simulink model "Noh_Nofusion"  (R2020b)
settings: Solver=FixedStepAuto  StartTime=0.0  StopTime=Inf  FixedStep=0.01  RelTol=1e-3
PostLoadFcn:
  | if any(exist('dsrtsu_mdlpostloadfcn', 'file') ~= 0), dsrtsu_mdlpostloadfcn('Execute', bdroot); end
InitFcn:
  | , if any(exist('rtifpga_mdlclblib', 'file') ~= 0), rtifpga_mdlclblib('Init', bdroot); end,
  | , if any(exist('dsmpb_private', 'file') ~= 0), dsmpb_private('dsmpb_mdlclblib', 'Init', bdroot); end,
undefined symbols (not defined in the file): ACC_TimeGap_DecSetSwt, ACC_TimeGap_IncSetSwt, AccelPedalPosn, AccelPedalPosnVldty, AccelPedlPosnDiagc, AccPedalOverride, ACU_ShiftInProgress, ADAS_Posn_CurLane, AESSwtReq, ALC_SwtReq, BrkPedalSts, CC_ACC_CANCEL_OFFSwt, CC_ACC_CRUISE_OFFSwt, CC_ACC_DecSetSpd_SetSwt, CC_ACC_IncSetSpd_ResuSwt, CC_ACCSwtErr, CharSpd_ms, CSA_NODE, CURRENT_GEAR, CurrentGearValid, DiscIntNeverNeededParam, DrvDoorSts, DrvSBR, DrvTrqReqOvld, ECMACCInterface, ECMRespACC, ELKSwtReq, EngLimpHomeSts, EngSpd, EngState, EngState_PHEV, EngTrqMaxActSpd, EngTrqMinAct, EPS_DrvInpTrqVal_HighReslolution, EPS_FailSts, EPS_LKATorqOvrlDlvd, EPS_LKATorqOvrlDlvdVld, EPS_LKATrqOvlDlvdSts, EPS_SteerMod, EPS_TrqSnsrSts, EQ4_APPINFO, EQ4_LA_ELEM, EQ4_LA_HDR, EQ4_LAP_ELEM, EQ4_LAP_HDR, EQ4_LH_ELEM, EQ4_LH_HDR, EQ4_LRE_ELEM, EQ4_LRE_HDR, ESS_PedSwtReq, ESS_VehSwtReq, FFogLmpSts_F_Pbox, FLWheelDriveDirection, FLWheelSpd, FrntWiprSwtSts, FrntWshrSwtSts, FRWheelDriveDirection, FRWheelSpd, HazardLmpSwtSts, HCU_AccelPedalPosn_Diag ... (+153)
libraries: simulink x132, dsmpblib x27
(part 8 of 14)

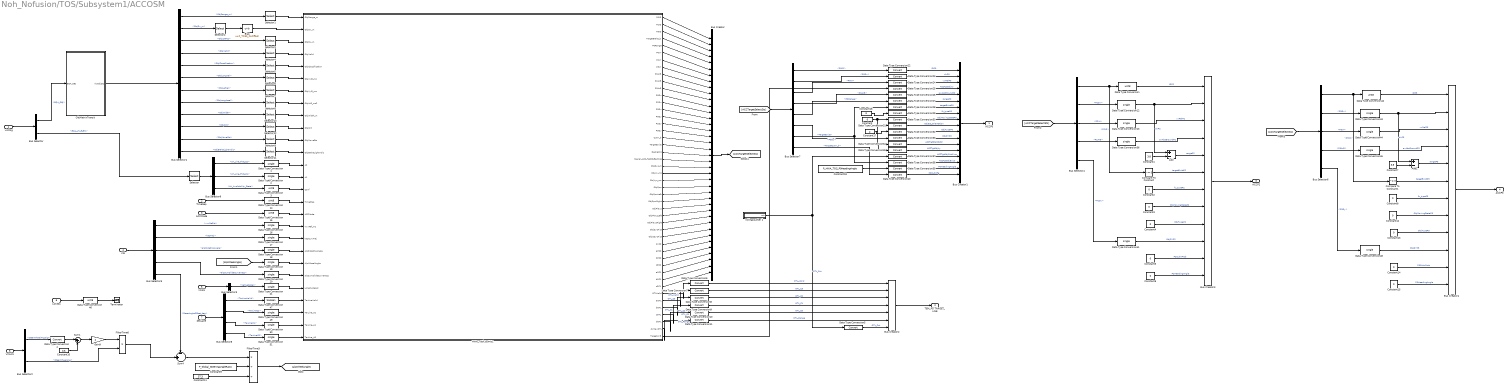
== system Noh_Nofusion/TOS/Subsystem1/ACCOSM ==
  visMsg : Inport
  TimeGap : Inport  Port=2
  ACCMode : Inport  Port=3
  VIE : Inport  Port=4
  VCAN : Inport  Port=5
  LCKSts : Inport  Port=6
  desLane : Inport  Port=7
  Add : Sum  Inputs=+-
  Add1 : Sum  Inputs=+-
  Bias : Bias  Bias=P_TOSS_DxOffset
  Bus Creator : BusCreator  Inputs=39
  Bus Creator1 : BusCreator  Inputs=18  OutDataTypeStr=Bus: TOS_ACCP0_BUS  NonVirtualBus=on
  Bus Creator2 : BusCreator  Inputs=7  OutDataTypeStr=Bus: TOS_P0_TARGET_LINE_BUS  NonVirtualBus=on
  Bus Creator3 : BusCreator  Inputs=12  OutDataTypeStr=Bus: TOS_ACCP2_BUS  NonVirtualBus=on
  Bus Creator4 : BusCreator  Inputs=12  OutDataTypeStr=Bus: TOS_ACCP3_BUS  NonVirtualBus=on
  Bus Selector : BusSelector  OutputSignals=EQ4_OBJ,EQ4_LH.EQ4_LH_ELEM
  Bus Selector4 : BusSelector  OutputSignals=P2ID,P2Dx,P2Vr,P2ArG,P2Dy
  Bus Selector6 : BusSelector  OutputSignals=P3ID,P3Dx,P3Vr,P3ArG,P3Dy
  Bus Selector7 : BusSelector  OutputSignals=P0ID,P0Dx,P0Vr,P0ArG,P0Range,P0Dy,TargetExist,TargetCutIn_b
  Bus Selector9 : BusSelector  OutputSignals=LH_Line_First_C2,LH_Line_First_C1,LH_Availability_State
  Bus Selector1 : BusSelector  OutputSignals=ObjRange_m,ObjDx_m,ObjLatPos,ObjValid,ObjClassification,ObjLongVel,ObjLatVel,ObjLongAccel,ObjWidth,ObjCnt,ObjMoveSts,ObjBrakeLightIndic
  Bus Selector2 : BusSelector  OutputSignals=CSA_NODE.CSA2_MSG.SteerWheelAngSign,CSA_NODE.CSA2_MSG.SteerWheelAng
  Bus Selector3 : BusSelector  OutputSignals=ABM_NODE.ABM2_MSG.VehLgtAccel
  Bus Selector5 : BusSelector  OutputSignals=vxvRefMs,kapTraj,alpSideSlipAngle,alpSumSlideCurveness,SteerAngleOffset_deg
  Bus Selector8 : BusSelector  OutputSignals=TarLineValid,TarLineC2,TarLineC1,TarLineC0
  Compare To Constant : simulink/Logic and Bit Operations/Compare To Constant  relop=~=  const=0  OutDataTypeStr=boolean
  Compare To Constant1 : simulink/Logic and Bit Operations/Compare To Constant  relop=~=  const=0  OutDataTypeStr=boolean
  Constant : Constant  Value=0
  Constant1 : Constant  Value=3.8  OutDataTypeStr=single
  Constant10 : Constant  Value=0.5  OutDataTypeStr=single
  Constant11 : Constant  Value=57.3  OutDataTypeStr=single
  Constant{2..4,8,12..13} (6 alike) : Constant  Value=0  OutDataTypeStr=uint8
  Constant{5..6,14..15} (4 alike) : Constant  Value=0  OutDataTypeStr=single
  Constant16 : Constant  Value=3
  Constant17 : Constant  Value=2
  Constant18 : Constant  Value=P_HWA_TOS_P0HeadingAngle
  Constant7 : Constant  Value=3.8  OutDataTypeStr=single
  Constant9 : Constant  Value=P_Global_SteeringAngleRatio
  Data Type Conversion{,3,14..15,42,46} (6 alike) : DataTypeConversion  OutDataTypeStr=uint8
  Data Type Conversion{1..2,12..13,16..21,36,41,43..45,48..51} (19 alike) : DataTypeConversion  OutDataTypeStr=single
  Data Type Conversion{4..11,22..35,37..40} (26 alike) : DataTypeConversion
  Data Type Conversion47 : DataTypeConversion  OutDataTypeStr=boolean
  FilterTime3 : Product  Inputs=*//  RndMeth=Zero
  FilterTime6 : Product  Inputs=**  RndMeth=Zero
  Gain9 : Gain  Gain=2
  HWA_Task100ms1 : Subsystem
  ObjMatrixTransit : Subsystem
  Selector : Selector  InputPortWidth=2  IndexOptions=Index vector (dialog)  Indices=1  OutputSizes=1
  Selector{1..12} (12 alike) : Selector  InputPortWidth=20  IndexOptions=Index vector (dialog)  Indices=[1:15]  OutputSizes=1
  Sum1 : Sum  Inputs=|-+
  Sum4 : Sum  Inputs=-+|
  Terminator : Terminator
  VCAN1 : InportShadow  Port=5
  rollingcounter 1 : Subsystem
  ACCP0 : Outport  OutDataTypeStr=Bus: TOS_ACCP0_BUS
  TEM_P0_TARGET_LINE : Outport  Port=2  OutDataTypeStr=Bus: TOS_P0_TARGET_LINE_BUS  PortDimensions=1  BusOutputAsStruct=on
  ACCP2 : Outport  Port=3  OutDataTypeStr=Bus: TOS_ACCP2_BUS
  ACCP3 : Outport  Port=4  OutDataTypeStr=Bus: TOS_ACCP3_BUS
  wires:
  Data Type Conversion51/1 -> HWA_Task100ms1/27(TarLine_A0)
  Data Type Conversion46/1 -> Terminator/1
  Constant18/1 -> Data Type Conversion39/1
  HWA_Task100ms1/46(TargetVyG) -> Data Type Conversion25/1
  Constant17/1 -> Data Type Conversion32/1
  Constant16/1 -> Data Type Conversion29/1
  Selector2/1 -> Bias/1
  [ACCTargetSelectSts] -> Bus Selector6/1
  Bus Selector6/1 -> Compare To Constant1/1, Data Type Conversion42/1  "<P3ID>"
  Data Type Conversion42/1 -> Bus Creator4/1  "IDP3"
  Bus Selector6/2 -> Data Type Conversion43/1  "<P3Dx>"
  Data Type Conversion43/1 -> Add1/1, Bus Creator4/2  "dxP3"
  Bus Selector6/3 -> Data Type Conversion44/1  "<P3Vr>"
  Data Type Conversion44/1 -> Bus Creator4/3  "vxRelP3"
  Bus Selector6/4 -> Data Type Conversion45/1  "<P3ArG>"
  Data Type Conversion45/1 -> Bus Creator4/4  "axAbsGroundP3"
  Add1/1 -> Bus Creator4/5  "rangeP3"
  Constant7/1 -> Add1/2
  Compare To Constant1/1 -> Bus Creator4/6  "targetExistP3"
  Constant8/1 -> Bus Creator4/7  "fu_typeP3"
  Constant12/1 -> Bus Creator4/8  "ObjMovingStateP3"
  Constant13/1 -> Bus Creator4/9  "ObjTypeP3"
  Bus Selector6/5 -> Data Type Conversion48/1  "<P3Dy>"
  Data Type Conversion48/1 -> Bus Creator4/10  "ObjDYP3"
  Constant14/1 -> Bus Creator4/11  "P3CutinProb"
  Constant15/1 -> Bus Creator4/12  "P3HeadingAngle"
  Bus Creator4/1 -> ACCP3/1
  Bus Creator3/1 -> ACCP2/1
  Constant6/1 -> Bus Creator3/12  "P2HeadingAngle"
  Constant5/1 -> Bus Creator3/11  "P2CutinProb"
  Data Type Conversion41/1 -> Bus Creator3/10  "ObjDYP2"
  Bus Selector4/5 -> Data Type Conversion41/1  "<P2Dy>"
  Constant4/1 -> Bus Creator3/9  "ObjTypeP2"
  Constant3/1 -> Bus Creator3/8  "ObjMovingStateP2"
  Constant2/1 -> Bus Creator3/7  "fu_typeP2"
  Compare To Constant/1 -> Bus Creator3/6  "targetExistP2"
  Constant1/1 -> Add/2
  Add/1 -> Bus Creator3/5  "rangeP2"
  Data Type Conversion36/1 -> Bus Creator3/4  "axAbsGroundP2"
  Bus Selector4/4 -> Data Type Conversion36/1  "<P2ArG>"
  Data Type Conversion13/1 -> Bus Creator3/3  "vxRelP2"
  Bus Selector4/3 -> Data Type Conversion13/1  "<P2Vr>"
  Data Type Conversion12/1 -> Bus Creator3/2, Add/1  "dxP2"
  Bus Selector4/2 -> Data Type Conversion12/1  "<P2Dx>"
  Data Type Conversion/1 -> Bus Creator3/1  "IDP2"
  Bus Selector4/1 -> Data Type Conversion/1, Compare To Constant/1  "<P2ID>"
  [ACCTargetSelectSts] -> Bus Selector4/1
  ObjMatrixTransit/1(VisObjSts) -> Bus Selector1/1
  Bus Selector/1 -> ObjMatrixTransit/1(EQ4_OBJ)  "<EQ4_OBJ>"
  Selector12/1 -> HWA_Task100ms1/10(ObjCnt)
  Selector11/1 -> HWA_Task100ms1/12(ObjBrakeLightIndic)
  Selector10/1 -> HWA_Task100ms1/9(ObjWidth_m)
  Selector9/1 -> HWA_Task100ms1/11(ObjMoveSts)
  Selector8/1 -> HWA_Task100ms1/8(ObjArG_ms2)
  Selector7/1 -> HWA_Task100ms1/7(ObjVyG_ms)
  Selector6/1 -> HWA_Task100ms1/6(ObjVxG_ms)
  Selector5/1 -> HWA_Task100ms1/5(ObjClassification)
  Selector4/1 -> HWA_Task100ms1/4(ObjValid)
  Selector3/1 -> HWA_Task100ms1/3(ObjDy_m)
  Bias/1 -> HWA_Task100ms1/2(ObjDx_m)
  Selector1/1 -> HWA_Task100ms1/1(ObjRange_m)
  Selector/1 -> Bus Selector9/1
  Bus Selector/2 -> Selector/1  "<EQ4_LH_ELEM>"
  visMsg/1 -> Bus Selector/1
  Data Type Conversion11/1 -> Bus Creator2/6  "OTL_Range"
  Data Type Conversion10/1 -> Bus Creator2/5  "OTL_C0"
  Data Type Conversion9/1 -> Bus Creator2/4  "OTL_C1"
  Data Type Conversion8/1 -> Bus Creator2/3  "OTL_C2"
  Data Type Conversion7/1 -> Bus Creator2/2  "OTL_C3"
  Data Type Conversion6/1 -> Bus Creator2/1  "OTL_Valid"
  Data Type Conversion5/1 -> Bus Creator2/7  "OTL_Cnt"
  Bus Creator2/1 -> TEM_P0_TARGET_LINE/1
  HWA_Task100ms1/42(bOTL) -> Data Type Conversion8/1  "OTL_C2"
  HWA_Task100ms1/41(aOTL) -> Data Type Conversion7/1  "OTL_C3"
  HWA_Task100ms1/40(OTLValid) -> Data Type Conversion6/1  "OTL_Valid"
  HWA_Task100ms1/43(cOTL) -> Data Type Conversion9/1  "OTL_C1"
  rollingcounter 1/1(cnt) -> Data Type Conversion5/1, Data Type Conversion37/1  "OTL_Cnt"
  HWA_Task100ms1/45(dxMaxOTL) -> Data Type Conversion11/1  "OTL_Range"
  HWA_Task100ms1/44(dOTL) -> Data Type Conversion10/1  "OTL_C0"
  Data Type Conversion4/1 -> Sum1/1
  Bus Selector2/2 -> FilterTime6/2  "<SteerWheelAng>"
  Bus Selector2/1 -> Data Type Conversion4/1  "<SteerWheelAngSign>"
  Sum1/1 -> Gain9/1
  Gain9/1 -> FilterTime6/1
  Constant10/1 -> Sum1/2
  VCAN1/1 -> Bus Selector2/1
  Constant9/1 -> FilterTime3/2
  Bus Selector5/5 -> Sum4/1  "<SteerAngleOffset_deg>"
  FilterTime3/1 -> [alpWheelAngle]
  Sum4/1 -> FilterTime3/1
  Constant11/1 -> FilterTime3/3
  FilterTime6/1 -> Sum4/2
  HWA_Task100ms1/34(aPC0) -> Bus Creator/34
  HWA_Task100ms1/38(bPC1) -> Bus Creator/38
  Bus Selector7/1 -> Data Type Conversion22/1  "<P0ID>"
  Data Type Conversion3/1 -> HWA_Task100ms1/15(Conf)
  Data Type Conversion22/1 -> Bus Creator1/1  "IDP0"
  Data Type Conversion27/1 -> Bus Creator1/6  "rangeP0"
  Data Type Conversion1/1 -> HWA_Task100ms1/13(A2)
  HWA_Task100ms1/2(P2ID) -> Bus Creator/2
  Data Type Conversion2/1 -> HWA_Task100ms1/14(A1)
  Data Type Conversion37/1 -> Bus Creator1/15  "ACCTgtObjCntAlive"
  HWA_Task100ms1/1(P0ID) -> Bus Creator/1
  Bus Selector3/1 -> Data Type Conversion21/1  "<VehLgtAccel>"
  Bus Selector1/9 -> Selector10/1  "<ObjWidth>"
  Data Type Conversion19/1 -> HWA_Task100ms1/21(AlpWheelAngle)
  Bus Selector7/3 -> Data Type Conversion24/1  "<P0Vr>"
  Bus Selector9/1 -> Data Type Conversion1/1  "<LH_Line_First_C2>"
  VIE/1 -> Bus Selector5/1
  Data Type Conversion38/1 -> Bus Creator1/16  "ACCTgtObjExist"
  Bus Selector7/6 -> Data Type Conversion33/1  "<P0Dy>"
  Bus Selector7/2 -> Data Type Conversion23/1  "<P0Dx>"
  Data Type Conversion29/1 -> Bus Creator1/8  "fu_typeP0"
  Bus Selector7/8 -> Data Type Conversion40/1  "<TargetCutIn_b>"
  HWA_Task100ms1/32(ObjqDycHist) -> Bus Creator/32
  Data Type Conversion32/1 -> Bus Creator1/11  "ObjTypeP0"
  Data Type Conversion35/1 -> Bus Creator1/14  "ACCTgtObjAy"
  VCAN/1 -> Bus Selector3/1
  Data Type Conversion34/1 -> Bus Creator1/13  "ACCTgtObjObstcl"
  Bus Selector8/1 -> Data Type Conversion47/1  "<TarLineValid>"
  Bus Selector5/1 -> Data Type Conversion16/1  "<vxvRefMs>"
  Data Type Conversion17/1 -> HWA_Task100ms1/19(kapCurvTraj)
  Data Type Conversion28/1 -> Bus Creator1/7  "targetExistP0"
  Bus Selector1/7 -> Selector7/1  "<ObjLatVel>"
  HWA_Task100ms1/8(P3Vr) -> Bus Creator/8
  Bus Selector1/8 -> Selector8/1  "<ObjLongAccel>"
  Data Type Conversion49/1 -> HWA_Task100ms1/25(TarLine_A2)
  ACCMode/1 -> Data Type Conversion15/1
  HWA_Task100ms1/22(ObjDyc_m) -> Bus Creator/22
  Data Type Conversion18/1 -> HWA_Task100ms1/20(AlpSideSlipAngle)
  Data Type Conversion30/1 -> Bus Creator1/9  "ObjMovingStateP0"
  HWA_Task100ms1/11(P3ArG) -> Bus Creator/11
  Data Type Conversion25/1 -> Bus Creator1/4  "ACCTgtObjVy"
  TimeGap/1 -> Data Type Conversion14/1
  Data Type Conversion23/1 -> Bus Creator1/2  "dxP0"
  Data Type Conversion21/1 -> HWA_Task100ms1/23(LongitudeAcc)
  Bus Creator/1 -> [ACCTargetSelectSts]
  HWA_Task100ms1/31(ObjDycHist) -> Bus Creator/31
  Bus Selector1/5 -> Selector5/1  "<ObjClassification>"
  Bus Selector7/5 -> Data Type Conversion27/1  "<P0Range>"
  Bus Selector5/2 -> Data Type Conversion17/1  "<kapTraj>"
  Bus Selector1/3 -> Selector3/1  "<ObjLatPos>"
  Constant/1 -> Data Type Conversion30/1, Data Type Conversion31/1, Data Type Conversion34/1, Data Type Conversion35/1
  Data Type Conversion47/1 -> HWA_Task100ms1/24(TarLineValid)
  HWA_Task100ms1/4(TargetBrake_b) -> Bus Creator/4
  Data Type Conversion14/1 -> HWA_Task100ms1/16(TimeGap)
  HWA_Task100ms1/15(P0Dy) -> Bus Creator/15
  HWA_Task100ms1/33(dxC0) -> Bus Creator/33
  Data Type Conversion39/1 -> Bus Creator1/17  "P0HeadingAngle"
  HWA_Task100ms1/21(Signal_ACC_TgtObjBarDisp) -> Bus Creator/21
  HWA_Task100ms1/24(ObjVyc_ms) -> Bus Creator/24
  HWA_Task100ms1/16(P2Dy) -> Bus Creator/16
  Bus Selector8/3 -> Data Type Conversion50/1  "<TarLineC1>"
  HWA_Task100ms1/30(ObjPlausRight) -> Bus Creator/30
  HWA_Task100ms1/13(P2Dx) -> Bus Creator/13
  Bus Selector1/11 -> Selector9/1  "<ObjMoveSts>"
  HWA_Task100ms1/35(bPC0) -> Bus Creator/35
  Data Type Conversion16/1 -> HWA_Task100ms1/18(VxvRef_ms)
  Bus Selector9/2 -> Data Type Conversion2/1  "<LH_Line_First_C1>"
  HWA_Task100ms1/18(CutIn_b) -> Bus Creator/18
  HWA_Task100ms1/27(ObjSpwRight) -> Bus Creator/27
  [ACCTargetSelectSts] -> Bus Selector7/1
  HWA_Task100ms1/3(P3ID) -> Bus Creator/3
  HWA_Task100ms1/20(DesireDis) -> Bus Creator/20
  Bus Selector7/4 -> Data Type Conversion26/1  "<P0ArG>"
  Data Type Conversion31/1 -> Bus Creator1/10  "Object_Orientation"
  Data Type Conversion50/1 -> HWA_Task100ms1/26(TarLine_A1)
  Bus Selector1/1 -> Selector1/1  "<ObjRange_m>"
  Bus Selector1/6 -> Selector6/1  "<ObjLongVel>"
  Bus Selector1/12 -> Selector11/1  "<ObjBrakeLightIndic>"
  Bus Selector5/3 -> Data Type Conversion18/1  "<alpSideSlipAngle>"
  HWA_Task100ms1/14(P3Dx) -> Bus Creator/14
  Data Type Conversion33/1 -> Bus Creator1/12  "ObjDYP0"
  Bus Selector5/4 -> Data Type Conversion20/1  "<alpSumSlideCurveness>"
  HWA_Task100ms1/9(P0ArG) -> Bus Creator/9
  HWA_Task100ms1/36(cPC0) -> Bus Creator/36
  HWA_Task100ms1/39(cPC1) -> Bus Creator/39
  HWA_Task100ms1/12(P0Dx) -> Bus Creator/12
  HWA_Task100ms1/17(P3Dy) -> Bus Creator/17
  HWA_Task100ms1/19(TargetExist) -> Bus Creator/19
  Bus Selector1/10 -> Selector12/1  "<ObjCnt>"
  HWA_Task100ms1/10(P2ArG) -> Bus Creator/10
  HWA_Task100ms1/26(ObjSpwLeft) -> Bus Creator/26
  HWA_Task100ms1/37(aPC1) -> Bus Creator/37
  HWA_Task100ms1/5(P0Range) -> Bus Creator/5
  Data Type Conversion26/1 -> Bus Creator1/5  "axAbsGroundP0"
  Bus Selector1/2 -> Selector2/1  "<ObjDx_m>"
  HWA_Task100ms1/28(ObjPlaus) -> Bus Creator/28
  LCKSts/1 -> Data Type Conversion46/1
  Data Type Conversion24/1 -> Bus Creator1/3  "vxRelP0"
  Bus Selector8/2 -> Data Type Conversion49/1  "<TarLineC2>"
  Bus Selector1/4 -> Selector4/1  "<ObjValid>"
  HWA_Task100ms1/7(P2Vr) -> Bus Creator/7
  HWA_Task100ms1/29(ObjPlausLeft) -> Bus Creator/29
  Data Type Conversion40/1 -> Bus Creator1/18  "P0CutInflg"
  desLane/1 -> Bus Selector8/1
  Bus Selector9/3 -> Data Type Conversion3/1  "<LH_Availability_State>"
  [alpWheelAngle] -> Data Type Conversion19/1
  HWA_Task100ms1/25(ObjSpw) -> Bus Creator/25
  HWA_Task100ms1/6(P0Vr) -> Bus Creator/6
  Bus Selector7/7 -> Data Type Conversion38/1, Data Type Conversion28/1  "<TargetExist>"
  Data Type Conversion15/1 -> HWA_Task100ms1/17(ACCMode)
  HWA_Task100ms1/23(ObjVy_ms) -> Bus Creator/23
  Data Type Conversion20/1 -> HWA_Task100ms1/22(alpSumSlideCurveness)
  Bus Selector8/4 -> Data Type Conversion51/1  "<TarLineC0>"
  Bus Creator1/1 -> ACCP0/1

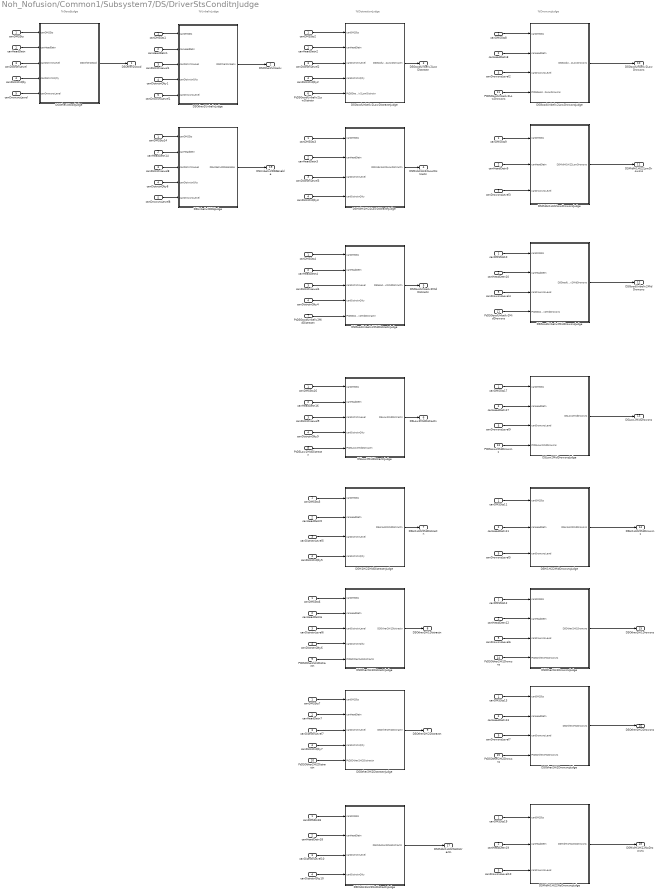
== system Noh_Nofusion/Common1/Subsystem7/DS/DriverStsConditnJudge ==
  note: %DrowsnsJudge
  note: %DistractionJudge
  note: %UnbelivJudge
  note: %GoodJudge
  canDMSSts : Inport
  canHeadDetn : Inport  Port=2
  canDistrctnLevel : Inport  Port=3
  canDistrctnQlty : Inport  Port=4
  canDrowsnsLevel : Inport  Port=5
  PtDSGoodUnbeliv2LowDistrctn : Inport  Port=6
  PtDSGoodUnbeliv2MidDistractn : Inport  Port=7
  PtDSLow2MidDistractn : Inport  Port=8
  PtDSOther2Hi1Distractn : Inport  Port=9
  PtDSOther2Hi2Distractn : Inport  Port=10
  PtDSGoodUnbeliv2LowDrowsns : Inport  Port=11
  PtDSGoodUnbeliv2MidDrowsns : Inport  Port=12
  PtDSLow2MidDrowsns : Inport  Port=13
  PtDSOther2Hi1Drowsns : Inport  Port=14
  PtDSOther2Hi2Drowsns : Inport  Port=15
  DSGoodUnbeliv2LowDistractnJudge : Subsystem
  DSGoodUnbeliv2LowDrowsnsJudge : Subsystem
  DSGoodUnbeliv2MidDistractnJudge : Subsystem
  DSGoodUnbeliv2MidDrowsnsJudge : Subsystem
  DSHi1Hi22MidDistractnJudge : Subsystem
  DSHi1Hi22MidDrowsnsJudge : Subsystem
  DSLow2MidDistractnJudge : Subsystem
  DSLow2MidDrowsnsJudge : Subsystem
  DSMidHi1Hi22LowDistractnJudge : Subsystem
  DSMidHi1Hi22LowDrowsnsJudge : Subsystem
  DSMidHi1Hi22NoDistractnJudge : Subsystem
  DSMidHi1Hi22NoDrowsnsJudge : Subsystem
  DSOther2GoodJudge : Subsystem
  DSOther2Hi1DistractnJudge : Subsystem
  DSOther2Hi1DrowsnsJudge : Subsystem
  DSOther2Hi2DistractnJudge : Subsystem
  DSOther2Hi2DrowsnsJudge : Subsystem
  DSOther2UnbelivJudge : Subsystem
  DSUnbeliv2DDAJudge : Subsystem
  canDMSSts{1..14,16..19} (18 alike) : InportShadow
  canDistrctnLevel{1..10} (10 alike) : InportShadow  Port=3
  canDistrctnQlty{1..10} (10 alike) : InportShadow  Port=4
  canDrowsnsLevel{1..10} (10 alike) : InportShadow  Port=5
  canHeadDetn{1..14,16..19} (18 alike) : InportShadow  Port=2
  DSOther2Good : Outport
  DSOther2Unbeliv : Outport  Port=2
  DSGoodUnbeliv2LowDistractn : Outport  Port=3
  DSMidHi1Hi22LowDistractn : Outport  Port=4
  DSGoodUnbeliv2MidDistractn : Outport  Port=5
  DSLow2MidDistractn : Outport  Port=6
  DSHi1Hi22MidDistractn : Outport  Port=7
  DSOther2Hi1Distractn : Outport  Port=8
  DSOther2Hi2Distractn : Outport  Port=9
  DSGoodUnbeliv2LowDrowsns : Outport  Port=10
  DSMidHi1Hi22LowDrowsns : Outport  Port=11
  DSGoodUnbeliv2MidDrowsns : Outport  Port=12
  DSLow2MidDrowsns : Outport  Port=13
  DSHi1Hi22MidDrowsns : Outport  Port=14
  DSOther2Hi1Drowsns : Outport  Port=15
  DSOther2Hi2Drowsns : Outport  Port=16
  DSMidHi1Hi22NoDistractn : Outport  Port=17
  DSMidHi1Hi22NoDrowsns : Outport  Port=18
  DSUnbeliv2DDAEnable : Outport  Port=19
  wires:
  PtDSOther2Hi2Drowsns/1 -> DSOther2Hi2DrowsnsJudge/4(PtDSOther2Hi2Drowsns)
  PtDSOther2Hi1Drowsns/1 -> DSOther2Hi1DrowsnsJudge/4(PtDSOther2Hi1Drowsns)
  PtDSLow2MidDrowsns/1 -> DSLow2MidDrowsnsJudge/4(PtDSLow2MidDrowsns)
  PtDSGoodUnbeliv2MidDrowsns/1 -> DSGoodUnbeliv2MidDrowsnsJudge/4(PtDSGoodUnbeliv2MidDrowsns)
  PtDSGoodUnbeliv2LowDrowsns/1 -> DSGoodUnbeliv2LowDrowsnsJudge/4(PtDSGoodUnbeliv2LowDrowsns)
  PtDSOther2Hi2Distractn/1 -> DSOther2Hi2DistractnJudge/5(PtDSOther2Hi2Distractn)
  PtDSOther2Hi1Distractn/1 -> DSOther2Hi1DistractnJudge/5(PtDSOther2Hi1Distractn)
  PtDSLow2MidDistractn/1 -> DSLow2MidDistractnJudge/5(PtDSLow2MidDistractn)
  PtDSGoodUnbeliv2MidDistractn/1 -> DSGoodUnbeliv2MidDistractnJudge/5(PtDSGoodUnbeliv2MidDistractn)
  PtDSGoodUnbeliv2LowDistrctn/1 -> DSGoodUnbeliv2LowDistractnJudge/5(PtDSGoodUnbeliv2LowDistrctn)
  DSUnbeliv2DDAJudge/1(DSUnbeliv2DDAEnable) -> DSUnbeliv2DDAEnable/1
  canDMSSts14/1 -> DSUnbeliv2DDAJudge/1(canDMSSts)
  canHeadDetn14/1 -> DSUnbeliv2DDAJudge/2(canHeadDetn)
  canDistrctnLevel8/1 -> DSUnbeliv2DDAJudge/3(canDistrctnLevel)
  canDistrctnQlty8/1 -> DSUnbeliv2DDAJudge/4(canDistrctnQlty)
  canDrowsnsLevel8/1 -> DSUnbeliv2DDAJudge/5(canDrowsnsLevel)
  DSMidHi1Hi22NoDrowsnsJudge/1(DSMidHi1Hi22NoDrowsns) -> DSMidHi1Hi22NoDrowsns/1
  canDMSSts19/1 -> DSMidHi1Hi22NoDrowsnsJudge/1(canDMSSts)
  canHeadDetn19/1 -> DSMidHi1Hi22NoDrowsnsJudge/2(canHeadDetn)
  canDrowsnsLevel10/1 -> DSMidHi1Hi22NoDrowsnsJudge/3(canDrowsnsLevel)
  DSMidHi1Hi22NoDistractnJudge/1(DSMidHi1Hi22NoDistractn) -> DSMidHi1Hi22NoDistractn/1
  canDMSSts18/1 -> DSMidHi1Hi22NoDistractnJudge/1(canDMSSts)
  canHeadDetn18/1 -> DSMidHi1Hi22NoDistractnJudge/2(canHeadDetn)
  canDistrctnLevel10/1 -> DSMidHi1Hi22NoDistractnJudge/3(canDistrctnLevel)
  canDistrctnQlty10/1 -> DSMidHi1Hi22NoDistractnJudge/4(canDistrctnQlty)
  DSLow2MidDrowsnsJudge/1(DSLow2MidDrowsns) -> DSLow2MidDrowsns/1
  canDMSSts17/1 -> DSLow2MidDrowsnsJudge/1(canDMSSts)
  canHeadDetn17/1 -> DSLow2MidDrowsnsJudge/2(canHeadDetn)
  canDrowsnsLevel9/1 -> DSLow2MidDrowsnsJudge/3(canDrowsnsLevel)
  canDMSSts16/1 -> DSLow2MidDistractnJudge/1(canDMSSts)
  canHeadDetn16/1 -> DSLow2MidDistractnJudge/2(canHeadDetn)
  canDistrctnLevel9/1 -> DSLow2MidDistractnJudge/3(canDistrctnLevel)
  canDistrctnQlty9/1 -> DSLow2MidDistractnJudge/4(canDistrctnQlty)
  DSLow2MidDistractnJudge/1(DSLow2MidDistractn) -> DSLow2MidDistractn/1
  DSOther2Hi2DrowsnsJudge/1(DSOther2Hi2Drowsns) -> DSOther2Hi2Drowsns/1
  canDMSSts13/1 -> DSOther2Hi2DrowsnsJudge/1(canDMSSts)
  canHeadDetn13/1 -> DSOther2Hi2DrowsnsJudge/2(canHeadDetn)
  canDrowsnsLevel7/1 -> DSOther2Hi2DrowsnsJudge/3(canDrowsnsLevel)
  DSOther2Hi1DrowsnsJudge/1(DSOther2Hi1Drowsns) -> DSOther2Hi1Drowsns/1
  canDrowsnsLevel6/1 -> DSOther2Hi1DrowsnsJudge/3(canDrowsnsLevel)
  canHeadDetn12/1 -> DSOther2Hi1DrowsnsJudge/2(canHeadDetn)
  canDMSSts12/1 -> DSOther2Hi1DrowsnsJudge/1(canDMSSts)
  canDMSSts11/1 -> DSHi1Hi22MidDrowsnsJudge/1(canDMSSts)
  canHeadDetn11/1 -> DSHi1Hi22MidDrowsnsJudge/2(canHeadDetn)
  canDrowsnsLevel5/1 -> DSHi1Hi22MidDrowsnsJudge/3(canDrowsnsLevel)
  DSHi1Hi22MidDrowsnsJudge/1(DSHi1Hi22MidDrowsns) -> DSHi1Hi22MidDrowsns/1
  DSGoodUnbeliv2MidDrowsnsJudge/1(DSGoodUnbeliv2MidDrowsns) -> DSGoodUnbeliv2MidDrowsns/1
  canDrowsnsLevel4/1 -> DSGoodUnbeliv2MidDrowsnsJudge/3(canDrowsnsLevel)
  canHeadDetn10/1 -> DSGoodUnbeliv2MidDrowsnsJudge/2(canHeadDetn)
  canDMSSts10/1 -> DSGoodUnbeliv2MidDrowsnsJudge/1(canDMSSts)
  canDrowsnsLevel3/1 -> DSMidHi1Hi22LowDrowsnsJudge/3(canDrowsnsLevel)
  canHeadDetn9/1 -> DSMidHi1Hi22LowDrowsnsJudge/2(canHeadDetn)
  canDMSSts9/1 -> DSMidHi1Hi22LowDrowsnsJudge/1(canDMSSts)
  DSMidHi1Hi22LowDrowsnsJudge/1(DSMidHi1Hi22LowDrowsns) -> DSMidHi1Hi22LowDrowsns/1
  canDrowsnsLevel2/1 -> DSGoodUnbeliv2LowDrowsnsJudge/3(canDrowsnsLevel)
  canHeadDetn8/1 -> DSGoodUnbeliv2LowDrowsnsJudge/2(canHeadDetn)
  canDMSSts8/1 -> DSGoodUnbeliv2LowDrowsnsJudge/1(canDMSSts)
  DSGoodUnbeliv2LowDrowsnsJudge/1(DSGoodUnbeliv2LowDrowsns) -> DSGoodUnbeliv2LowDrowsns/1
  canDistrctnQlty7/1 -> DSOther2Hi2DistractnJudge/4(canDistrctnQlty)
  canDistrctnLevel7/1 -> DSOther2Hi2DistractnJudge/3(canDistrctnLevel)
  canHeadDetn7/1 -> DSOther2Hi2DistractnJudge/2(canHeadDetn)
  canDMSSts7/1 -> DSOther2Hi2DistractnJudge/1(canDMSSts)
  DSOther2Hi2DistractnJudge/1(DSOther2Hi2Distractn) -> DSOther2Hi2Distractn/1
  canDistrctnQlty6/1 -> DSOther2Hi1DistractnJudge/4(canDistrctnQlty)
  canDistrctnLevel6/1 -> DSOther2Hi1DistractnJudge/3(canDistrctnLevel)
  canHeadDetn6/1 -> DSOther2Hi1DistractnJudge/2(canHeadDetn)
  canDMSSts6/1 -> DSOther2Hi1DistractnJudge/1(canDMSSts)
  DSOther2Hi1DistractnJudge/1(DSOther2Hi1Distractn) -> DSOther2Hi1Distractn/1
  DSHi1Hi22MidDistractnJudge/1(DSHi1Hi22MidDistractn) -> DSHi1Hi22MidDistractn/1
  canDistrctnQlty5/1 -> DSHi1Hi22MidDistractnJudge/4(canDistrctnQlty)
  canDistrctnLevel5/1 -> DSHi1Hi22MidDistractnJudge/3(canDistrctnLevel)
  canHeadDetn5/1 -> DSHi1Hi22MidDistractnJudge/2(canHeadDetn)
  canDMSSts5/1 -> DSHi1Hi22MidDistractnJudge/1(canDMSSts)
  DSGoodUnbeliv2MidDistractnJudge/1(DSGoodUnbeliv2MidDistractn) -> DSGoodUnbeliv2MidDistractn/1
  canDistrctnQlty4/1 -> DSGoodUnbeliv2MidDistractnJudge/4(canDistrctnQlty)
  canDistrctnLevel4/1 -> DSGoodUnbeliv2MidDistractnJudge/3(canDistrctnLevel)
  canHeadDetn4/1 -> DSGoodUnbeliv2MidDistractnJudge/2(canHeadDetn)
  canDMSSts4/1 -> DSGoodUnbeliv2MidDistractnJudge/1(canDMSSts)
  DSMidHi1Hi22LowDistractnJudge/1(DSMidHi1Hi22LowDistractn) -> DSMidHi1Hi22LowDistractn/1
  canDistrctnQlty3/1 -> DSMidHi1Hi22LowDistractnJudge/4(canDistrctnQlty)
  canDistrctnLevel3/1 -> DSMidHi1Hi22LowDistractnJudge/3(canDistrctnLevel)
  canHeadDetn3/1 -> DSMidHi1Hi22LowDistractnJudge/2(canHeadDetn)
  canDMSSts3/1 -> DSMidHi1Hi22LowDistractnJudge/1(canDMSSts)
  canDistrctnQlty2/1 -> DSGoodUnbeliv2LowDistractnJudge/4(canDistrctnQlty)
  canDistrctnLevel2/1 -> DSGoodUnbeliv2LowDistractnJudge/3(canDistrctnLevel)
  canHeadDetn2/1 -> DSGoodUnbeliv2LowDistractnJudge/2(canHeadDetn)
  canDMSSts2/1 -> DSGoodUnbeliv2LowDistractnJudge/1(canDMSSts)
  DSGoodUnbeliv2LowDistractnJudge/1(DSGoodUnbeliv2LowDistractn) -> DSGoodUnbeliv2LowDistractn/1
  DSOther2UnbelivJudge/1(DSOther2Unbeliv) -> DSOther2Unbeliv/1
  canDrowsnsLevel1/1 -> DSOther2UnbelivJudge/5(canDrowsnsLevel)
  canDistrctnQlty1/1 -> DSOther2UnbelivJudge/4(canDistrctnQlty)
  canDistrctnLevel1/1 -> DSOther2UnbelivJudge/3(canDistrctnLevel)
  canHeadDetn1/1 -> DSOther2UnbelivJudge/2(canHeadDetn)
  canDMSSts1/1 -> DSOther2UnbelivJudge/1(canDMSSts)
  canDrowsnsLevel/1 -> DSOther2GoodJudge/5(canDrowsnsLevel)
  canDistrctnQlty/1 -> DSOther2GoodJudge/4(canDistrctnQlty)
  canDistrctnLevel/1 -> DSOther2GoodJudge/3(canDistrctnLevel)
  canHeadDetn/1 -> DSOther2GoodJudge/2(canHeadDetn)
  DSOther2GoodJudge/1(DSOther2Good) -> DSOther2Good/1
  canDMSSts/1 -> DSOther2GoodJudge/1(canDMSSts)

== system Noh_Nofusion/Subsystem2/ACCOSM/HWA_Task100ms1/OTL1 ==
  vRef : Inport
  tCycle : Inport  Port=2
  tSameHandle : Inport  Port=3
  CutIn : Inport  Port=4
  P0Dx : Inport  Port=5
  P0Dy : Inport  Port=6
  EgoDDeltaX : Inport  Port=7
  EgoDDeltaY : Inport  Port=8
  EgoCosOfPsi : Inport  Port=9
  EgoSinOfPsi : Inport  Port=10
  Memory31 : Memory  InitialCondition=zeros(24,1)  InheritSampleTime=on
  Memory32 : Memory  InitialCondition=zeros(24,1)  InheritSampleTime=on
  Memory33 : Memory  InitialCondition=uint8(0)  InheritSampleTime=on
  P0TrajHistCalc01 : MATLAB Function  TreatAsAtomicUnit=on
  P0TrajHistCalc1 : MATLAB Function  TreatAsAtomicUnit=on
  Terminator : Terminator
  Terminator1 : Terminator
  Terminator2 : Terminator
  LineValid : Outport
  a : Outport  Port=2
  b : Outport  Port=3
  c : Outport  Port=4
  d : Outport  Port=5
  dxMin : Outport  Port=6
  dxMax : Outport  Port=7
  wires:
  vRef/1 -> P0TrajHistCalc01/1(vRef)
  CutIn/1 -> P0TrajHistCalc01/4(CutIn)
  P0TrajHistCalc1/8(d) -> d/1
  P0TrajHistCalc1/10(dxMax) -> dxMax/1
  P0TrajHistCalc1/9(dxMin) -> dxMin/1
  P0TrajHistCalc1/7(c) -> c/1
  P0TrajHistCalc1/6(b) -> b/1
  P0TrajHistCalc1/5(a) -> a/1
  P0TrajHistCalc1/4(LineValid) -> LineValid/1
  P0TrajHistCalc1/3(P0TrajHistDyv) -> Terminator2/1
  P0TrajHistCalc1/2(P0TrajHistDxv) -> Terminator1/1
  P0TrajHistCalc1/1(P0TrajHistNum) -> Terminator/1
  P0Dy/1 -> P0TrajHistCalc01/6(P0Dy)
  P0Dx/1 -> P0TrajHistCalc01/5(P0Dx)
  tSameHandle/1 -> P0TrajHistCalc01/3(tSameHandle)
  EgoCosOfPsi/1 -> P0TrajHistCalc01/9(EgoCosOfPsi)
  tCycle/1 -> P0TrajHistCalc01/2(tCycle)
  Memory31/1 -> P0TrajHistCalc01/13(P0TrajHistDyvK1)
  EgoDDeltaY/1 -> P0TrajHistCalc01/8(EgoDDeltaY)
  P0TrajHistCalc01/2(P0TrajHistDxv) -> Memory32/1, P0TrajHistCalc1/2(P0TrajHistDxv1)
  Memory32/1 -> P0TrajHistCalc01/12(P0TrajHistDxvK1)
  P0TrajHistCalc01/1(P0TrajHistNum) -> Memory33/1, P0TrajHistCalc1/1(P0TrajHistNum1)
  EgoSinOfPsi/1 -> P0TrajHistCalc01/10(EgoSinOfPsi)
  Memory33/1 -> P0TrajHistCalc01/11(P0TrajHistNumK1)
  P0TrajHistCalc01/3(P0TrajHistDyv) -> Memory31/1, P0TrajHistCalc1/3(P0TrajHistDyv1)
  EgoDDeltaX/1 -> P0TrajHistCalc01/7(EgoDDeltaX)

== system Noh_Nofusion/Subsystem2/ACCOSM/HWA_Task100ms1/Trajectory ==
  Kap : Inport
  VxvRef : Inport  Port=2
  AlpSideSlipAngle : Inport  Port=3
  ObjValid : Inport  Port=4
  ObjDx : Inport  Port=5
  ObjDy : Inport  Port=6
  ObjClass : Inport  Port=7
  ObjCntAlive : Inport  Port=8
  Terminator{1,3..10} (9 alike) : Terminator
  Trajectory : Subsystem  mask{ObjNum=15, TrajNum=10, BufNum=24}
      mask prompts: ObjNum "ObjectNumber"; TrajNum "TrajectoryNumber"; BufNum "BufferNumber"
  Out8 : Outport
  Out9 : Outport  Port=2
  Out10 : Outport  Port=3
  Out11 : Outport  Port=4
  Out12 : Outport  Port=5
  Out13 : Outport  Port=6
  EgoMove : Outport  Port=7
  wires:
  Trajectory/16(EgoMove) -> EgoMove/1
  Trajectory/11(TrajHistBufferBValid) -> Out11/1
  Trajectory/12(TrajHistBufferDxv) -> Out12/1
  Trajectory/13(TrajHistBufferDyv) -> Out13/1
  ObjValid/1 -> Trajectory/4(ObjValid)
  ObjDx/1 -> Trajectory/5(ObjectDx)
  ObjDy/1 -> Trajectory/6(ObjectDy)
  ObjClass/1 -> Trajectory/7(ObjectClass)
  ObjCntAlive/1 -> Trajectory/8(ObjectCntAlive)
  Kap/1 -> Trajectory/1(KapTraj)
  Trajectory/8(TrajHistBufferBTrajEnd) -> Out8/1
  Trajectory/2(EgoTrajHistDxv) -> Terminator4/1
  Trajectory/5(ObjPrio) -> Terminator8/1
  Trajectory/1(EgoTrajHistCurrentIndex) -> Terminator3/1
  AlpSideSlipAngle/1 -> Trajectory/3(AlpSideSlipAngle)
  Trajectory/7(TrajUsed) -> Terminator9/1
  Trajectory/10(TrajCurrentIndex) -> Out10/1
  Trajectory/6(ObjMatrix) -> Terminator10/1
  Trajectory/4(EgoTrajHistTTimeStamp) -> Terminator7/1
  VxvRef/1 -> Trajectory/2(VxvRef)
  Trajectory/3(EgoTrajHistDyv) -> Terminator5/1
  Trajectory/9(ObjTrajNumber) -> Out9/1
  Trajectory/14(TrajHistBufferTTimeStamp) -> Terminator6/1
  Trajectory/15(TrajHistBufferClass) -> Terminator1/1

== system Noh_Nofusion/Subsystem2/ACCOSM/HWA_Task100ms1/VxVy ==
  VxvRef : Inport
  Kap : Inport  Port=2
  VxG : Inport  Port=3
  VyG : Inport  Port=4
  Constant2 : Constant  Value=P_Global_EQ2RearAxisX_m  OutDataTypeStr=single
  Constant4 : Constant  Value=SideSlipAnglefactor  OutDataTypeStr=single
  Divide11 : Product
  Divide3 : Product  Inputs=3
  Divide4 : Product
  Divide5 : Product
  Gain10 : Gain  Gain=-1
  Gain9 : Gain  Gain=-1
  Sum1 : Sum  Inputs=+-
  Sum10 : Sum  Inputs=+-|
  Sum11 : Sum  Inputs=|-+
  Trigonometric Function : Trigonometry  Operator=atan  OutputSignalType=real
  Trigonometric Function1 : Trigonometry  Operator=cos
  Trigonometric Function2 : Trigonometry
  Vx : Outport
  Vy : Outport  Port=2
  wires:
  VxvRef/1 -> Divide3/2, Divide11/1, Divide5/1, Divide3/3
  Constant4/1 -> Divide3/1
  Trigonometric Function/1 -> Gain9/1
  Divide11/1 -> Sum11/1
  Constant2/1 -> Sum1/1
  Trigonometric Function1/1 -> Divide5/2
  Divide4/1 -> Trigonometric Function/1
  Divide5/1 -> Sum10/2
  Gain10/1 -> Trigonometric Function1/1, Trigonometric Function2/1
  Divide3/1 -> Sum1/2
  [IFVMoveAngle] -> Gain10/1
  Trigonometric Function2/1 -> Divide11/2
  Sum1/1 -> Divide4/1
  Gain9/1 -> [IFVMoveAngle]
  VxG/1 -> Sum10/1
  Sum11/1 -> Vy/1  "Vy"
  Sum10/1 -> Vx/1  "Vx"
  VyG/1 -> Sum11/2
  Kap/1 -> Divide4/2

== system Noh_Nofusion/Subsystem2/ACCOSM/ObjMatrixTransit/Subsystem ==
  Count : Inport
  <EQ4_OBJ_ELEM> : Inport  Port=2
  Bus Creator : BusCreator  Inputs=12
  Bus Selector : BusSelector  OutputSignals=id,BrakeLight,classification,LatDis,AbsLatVel,AbsLongAcc,LongDis,AbsLongVel,width,Age,motionSts
  For Each Subsystem : Subsystem  TreatAsAtomicUnit=on
  For Iterator Subsystem : Subsystem  Commented=on  TreatAsAtomicUnit=on
  MATLAB Function1 : MATLAB Function  TreatAsAtomicUnit=on
  Obj : Stateflow chart  Commented=on  TreatAsAtomicUnit=on
  Terminator : Terminator
  Terminator1 : Terminator
  Unit Delay1 : UnitDelay  SampleTime=-1  HasFrameUpgradeWarning=on
  ObjID : Outport
  ObjValid : Outport  Port=2
  ObjBrakeLightIndic : Outport  Port=3
  ObjClassification : Outport  Port=4
  ObjLatPos : Outport  Port=5
  ObjLatVel : Outport  Port=6
  ObjLongAccel : Outport  Port=7
  ObjLongVel : Outport  Port=8
  ObjWidth : Outport  Port=9
  ObjCnt : Outport  Port=10
  ObjMoveSts : Outport  Port=11
  ObjLongPos : Outport  Port=12
  P : Outport  Port=13
  wires:
  MATLAB Function1/10(ObjCnt) -> ObjCnt/1
  MATLAB Function1/9(ObjWidth) -> ObjWidth/1
  MATLAB Function1/8(ObjLongVel) -> ObjLongVel/1
  MATLAB Function1/3(ObjBrakeLightIndic) -> ObjBrakeLightIndic/1
  MATLAB Function1/6(ObjLatVel) -> ObjLatVel/1
  MATLAB Function1/2(ObjValid) -> ObjValid/1
  <EQ4_OBJ_ELEM>/1 -> For Each Subsystem/1(<EQ4_OBJ_ELEM>)
  Unit Delay1/1 -> MATLAB Function1/13(ObjIDK1)
  Bus Selector/1 -> MATLAB Function1/2(ID)  "<id>"
  Bus Selector/2 -> MATLAB Function1/3(BrakeLight_b)  "<BrakeLight>"
  MATLAB Function1/1(P) -> P/1
  MATLAB Function1/12(ObjLongPos) -> ObjLongPos/1
  Bus Selector/11 -> MATLAB Function1/12(MotionSts)  "<motionSts>"
  MATLAB Function1/11(ObjMoveSts) -> ObjMoveSts/1
  Bus Selector/4 -> MATLAB Function1/5(LatDis)  "<LatDis>"
  Bus Selector/6 -> MATLAB Function1/7(LongAccel)  "<AbsLongAcc>"
  Bus Selector/5 -> MATLAB Function1/6(LatVel)  "<AbsLatVel>"
  Bus Selector/9 -> MATLAB Function1/10(Width)  "<width>"
  Bus Selector/7 -> MATLAB Function1/8(LongDis)  "<LongDis>"
  For Each Subsystem/2(confidence) -> Bus Creator/2  "confidence"
  For Each Subsystem/11(Age) -> Bus Creator/11  "Age"
  For Each Subsystem/1(id) -> Bus Creator/1  "id"
  Bus Selector/3 -> MATLAB Function1/4(Class)  "<classification>"
  Bus Selector/8 -> MATLAB Function1/9(LongVel)  "<AbsLongVel>"
  For Each Subsystem/3(classification) -> Bus Creator/3  "classification"
  Bus Selector/10 -> MATLAB Function1/11(Age)  "<Age>"
  For Each Subsystem/5(LongDis) -> Bus Creator/5  "LongDis"
  For Each Subsystem/9(AbsLatVel) -> Bus Creator/9  "AbsLatVel"
  For Each Subsystem/13(motionCategory) -> Terminator/1
  For Each Subsystem/4(width) -> Bus Creator/4  "width"
  For Each Subsystem/8(AbsLongVel) -> Bus Creator/8  "AbsLongVel"
  Count/1 -> MATLAB Function1/1(Count)
  For Each Subsystem/14(motionOrientation) -> Terminator1/1
  MATLAB Function1/7(ObjLongAccel) -> ObjLongAccel/1
  MATLAB Function1/4(ObjClassification) -> ObjClassification/1
  For Each Subsystem/12(motionSts) -> Bus Creator/12  "motionSts"
  For Each Subsystem/7(AbsLongAcc) -> Bus Creator/7  "AbsLongAcc"
  MATLAB Function1/5(ObjLatPos) -> ObjLatPos/1
  For Each Subsystem/10(BrakeLight) -> Bus Creator/10  "BrakeLight"
  MATLAB Function1/13(ObjID) -> Unit Delay1/1, ObjID/1  "ObjBrakeLightIndic"
  Bus Creator/1 -> Bus Selector/1
  For Each Subsystem/6(LatDis) -> Bus Creator/6  "LatDis"
